simulink model "Cubesat_Control_LQR"  (R2025b)
settings: Solver=ode45  StartTime=0.0  StopTime=t_stop  RelTol=1e-3
values from neighbouring files (symbols this model uses):
  J = 0.000634    [Matlab_to_BLE2.m]    (also in Run_CubeSat_HIL.m; init_simulation_lqr.m; init_simulation_pd.m = 0.002)
  Jw = 4.607e-5    (= 4.607e-05)    [Matlab_to_BLE2.m]    (also in Run_CubeSat_HIL.m; init_simulation_lqr.m; init_simulation_pd.m = 1e-05)
  Kd_detumble = 0.0003    [Matlab_to_BLE2.m]    (also in Run_CubeSat_HIL.m = 0.03; init_simulation_lqr.m = lqr(A_d, B_d, Q_d, R_d); init_simulation_pd.m = 0.03)
  Kp_lqr = lqr(A, B, Q, R)    [init_simulation_lqr.m]
  omega0 = deg2rad(omega0_deg)    [init_simulation_lqr.m]    (also in init_simulation_pd.m)
  omega_th_high = deg2rad(10)    [Run_CubeSat_HIL.m]    (also in init_simulation_lqr.m = deg2rad(10000); init_simulation_pd.m = deg2rad(10000))
  omega_th_low = deg2rad(2.0)    [Run_CubeSat_HIL.m]    (also in init_simulation_lqr.m = deg2rad(0.3); init_simulation_pd.m = deg2rad(0.3))
  omega_w0 = 0    [init_simulation_lqr.m]    (also in init_simulation_pd.m)
  tau_max = 0.002    [Matlab_to_BLE2.m]    (also in Run_CubeSat_HIL.m; analyze_multiple_experiments.m; init_simulation_lqr.m; init_simulation_pd.m)
  theta0 = theta(1)    [analyze_multiple_experiments.m]    (also in init_simulation_lqr.m = deg2rad(0); init_simulation_pd.m = deg2rad(0))
  theta_ref = deg2rad(theta_ref_deg)    [Matlab_to_BLE2.m]    (also in analyze_multiple_experiments.m = theta_ref_deg; init_simulation_lqr.m; init_simulation_pd.m)
settings Model: Creator=bbtp  LastModifiedBy=bbtp

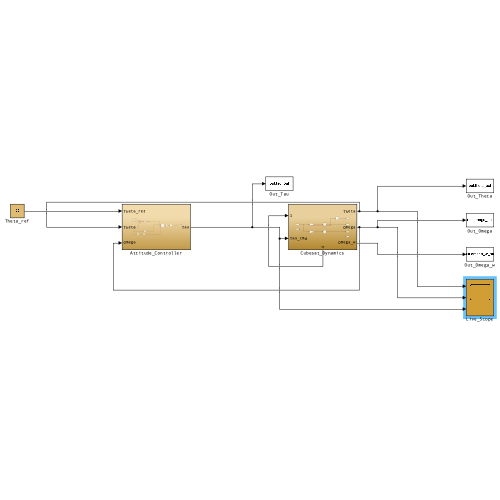
[thumbnail: Simulink's stored preview of the top-level diagram]
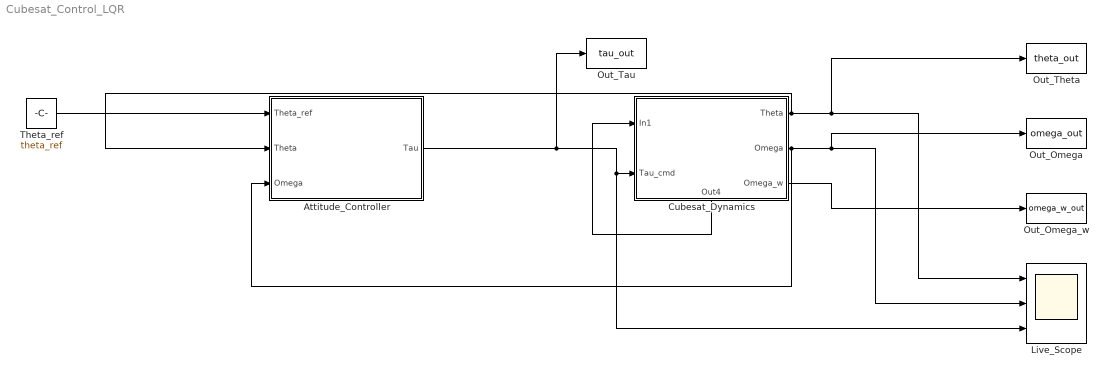
== system Cubesat_Control_LQR ==
  Attitude_Controller : Subsystem
  Cubesat_Dynamics : Subsystem
      settings: PortSchema="{\"entries\":[{\"content\":{\"sides\":[{\"content\":{\"connectorIds\":[\"In1\",\"In2\"]},\"type\":\"ConnectorPlacement.EquallySpacedRectSide\",\"uuid\":\"07d3b4e1-e370-42c3-b8dd-193f90ee50e1\"},{\"content\":{\"connectorIds\":[\"Out1\",\"Out2\",\"Out3\"],\"side\":\"RIGHT\"},\"type\":\"ConnectorPlacement.EquallySpacedRectSide\",\"uuid\":\"51b80ba3-acce-4020-bb7a-43983b3e1927\"},{\"content\":{\"side\":\"TOP\"},\"type\":\"ConnectorPlacement.EquallySpacedRectSide\",\"uuid\":\"242c82b8-16ac-45be-a9d2-cf3e89123009\"},{\"content\":{\"connectorIds\":[\"Out4\"],\"side\":\"BOTTOM\"},\"type\":\"ConnectorPlacement.EquallySpacedRectSide\",\"uuid\":\"a2422906-7725-4129-9f43-de2359fa30da\"}]},\"type\":\"ConnectorPlacement.EquallySpacedConnector\",\"uuid\":\"1c6cd9cc-95ea-45e9-9068-0a2498ad65e7\"}],\"packageUris\":[\"http://schema.mathworks.com/mf0/Connector/R2020b\"],\"version\":\"1.0\"}"
  Live_Scope : Scope  NumInputPorts=3
      settings: ActiveDisplayYMinimum=-0.394948893967831  ActiveDisplayYMaximum=3.53454004571048
  Out_Omega : ToWorkspace  VariableName=omega_out  SampleTime=-1
  Out_Omega_w : ToWorkspace  VariableName=omega_w_out  SampleTime=-1
  Out_Tau : ToWorkspace  VariableName=tau_out  SampleTime=-1
  Out_Theta : ToWorkspace  VariableName=theta_out  SampleTime=-1
  Theta_ref : Constant  Value=theta_ref
  wires:
  Theta_ref/1 -> Attitude_Controller/1(Theta_ref)
  Attitude_Controller/1(Tau) -> Cubesat_Dynamics/2(Tau_cmd), Live_Scope/3, Out_Tau/1
  Cubesat_Dynamics/1(Theta) -> Out_Theta/1, Live_Scope/1, Attitude_Controller/2(Theta)
  Cubesat_Dynamics/2(Omega) -> Out_Omega/1, Live_Scope/2, Attitude_Controller/3(Omega)
  Cubesat_Dynamics/3(Omega_w) -> Out_Omega_w/1
  Cubesat_Dynamics/4(Out4) -> Cubesat_Dynamics/1(In1)

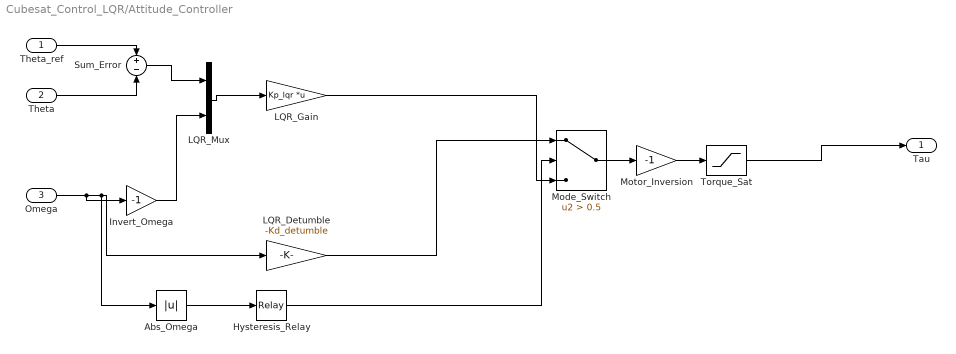
== system Cubesat_Control_LQR/Attitude_Controller ==
  Theta_ref : Inport
  Theta : Inport  Port=2
  Omega : Inport  Port=3
  Abs_Omega : Abs  SaturateOnIntegerOverflow=off
  Hysteresis_Relay : Relay  OnSwitchValue=omega_th_high  OffSwitchValue=omega_th_low
  Invert_Omega : Gain  Gain=-1
  LQR_Detumble : Gain  Gain=-Kd_detumble
  LQR_Gain : Gain  Gain=Kp_lqr  Multiplication=Matrix(K*u)
  LQR_Mux : Mux  Inputs=2
  Mode_Switch : Switch  Criteria=u2 > Threshold  Threshold=0.5  SaturateOnIntegerOverflow=off  InputSameDT=off
  Motor_Inversion : Gain  Gain=-1
  Sum_Error : Sum  Inputs=+-
  Torque_Sat : Saturate  UpperLimit=tau_max  LowerLimit=-tau_max
  Tau : Outport
  wires:
  ? -> ?
  Theta_ref/1 -> Sum_Error/1
  Theta/1 -> Sum_Error/2
  Sum_Error/1 -> LQR_Mux/1
  Omega/1 -> LQR_Detumble/1, Abs_Omega/1, Invert_Omega/1
  Invert_Omega/1 -> LQR_Mux/2
  LQR_Mux/1 -> LQR_Gain/1
  LQR_Detumble/1 -> Mode_Switch/1
  Abs_Omega/1 -> Hysteresis_Relay/1
  Hysteresis_Relay/1 -> Mode_Switch/2
  LQR_Gain/1 -> Mode_Switch/3
  Mode_Switch/1 -> Motor_Inversion/1
  Motor_Inversion/1 -> Torque_Sat/1
  Torque_Sat/1 -> Tau/1

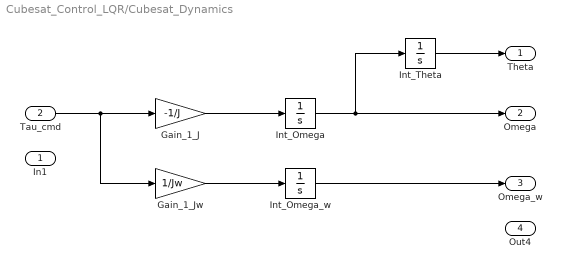
== system Cubesat_Control_LQR/Cubesat_Dynamics ==
  In1 : Inport
  Tau_cmd : Inport  Port=2
  Gain_1_J : Gain  Gain=-1/J
  Gain_1_Jw : Gain  Gain=1/Jw
  Int_Omega : Integrator  InitialCondition=omega0
  Int_Omega_w : Integrator  InitialCondition=omega_w0
  Int_Theta : Integrator  InitialCondition=theta0
  Theta : Outport
  Omega : Outport  Port=2
  Omega_w : Outport  Port=3
  Out4 : Outport  Port=4
  wires:
  ? -> ?
  Tau_cmd/1 -> Gain_1_Jw/1, Gain_1_J/1
  Gain_1_Jw/1 -> Int_Omega_w/1
  Gain_1_J/1 -> Int_Omega/1
  Int_Omega/1 -> Int_Theta/1, Omega/1
  Int_Theta/1 -> Theta/1
  Int_Omega_w/1 -> Omega_w/1
